simulink model "optotrak_double_pendulum_and_VR_v2"  (R2019b)
settings: Solver=ode3  StartTime=0.0  StopTime=inf  FixedStep=0.01  RelTol=1e-3  EnableMultiTasking=on
libraries: mblibv1 x4, xpcrtudplib x2, xpcutilitieslib x2, vrlib x2, slrtlib x1
(part 2 of 2)

== matlab function optotrak_double_pendulum_and_VR_v2/Embedded MATLAB Function1 ==
  data: R output; T1 input; T2 input
function R=R_iz_markerjev(T1,T2)
% Roman Kamnik, avgust 2010


%  Orientacijaska matrika segmenta iz markerjev.
%



%  H matrika pripeta na segment - lokalni ks
% osi koordinatenga sistema



tmp =  [0;0;1];
yos = unit(T1-T2);
xos = unit(cross(yos,tmp));
zos = unit(cross(xos, yos));

RR = [xos yos zos];

 
R = [RR(1,1); RR(2,1); RR(3,1); RR(1,2); RR(2,2); RR(3,2); RR(1,3); RR(2,3); RR(3,3)]; 
 
return;



%%%%%%%%%%%%%%%%%%%%%%%%%%%%%%%%%%%%%%%%%%%%%%%%%%%%%%%%%%%%%%%%%%%%%%%%

function u = unit(v)
	%u = v / norm(v,'fro');
    u = v / norm(v,2);
return    

% %%%%%%%%%%%%%%%%%%%%%%%%%%%%%%%%%%%%%%%%%%%%%%%%%%%%%%%%%%%%%%%%%%%%%%%%%

== matlab function optotrak_double_pendulum_and_VR_v2/Embedded MATLAB Function8 ==
  data: M1 input; COM output; M2 input
function COM= COM(M1, M2) 
% This block supports the Embedded MATLAB subset.
% See the help menu for details. 


d = 0.045;


C1 = M1;
C2 = M2;

COM = C1;



  
return;


%%%%%%%%%%%%%%%%%%%%%%%%%%%%%%%%%%%%%%%%%%%%%%%%%%%%%%%%%%%%%%%%%%%%%%%%

function u = unit(v)
	%u = v / norm(v,'fro');
    u = v / norm(v,2);
return    

% %%%%%%%%%%%%%%%%%%%%%%%%%%%%%%%%%%%%%%%%%%%%%%%%%%%%%%%%%%%%%%%%%%%%%%%%%

== matlab function optotrak_double_pendulum_and_VR_v2/Embedded MATLAB Function10 ==
  data: R1_in input size=[9 1]; X2 output; R2_in input size=[9 1]
function X2  = fcn1(R1_in,R2_in)
% This block supports the Embedded MATLAB subset.
% See the help menu for details. 


% Transformacija iz lokalnih ks segmentov v SimMech v lokalne ks segmentov v VR modelu
% columnwise as a 9-component row vector: (R11,  R21, R31,  R12, ... ).

% dolocitev orientacijske matrike med dvema segmentoma v vr, ce poznam R matriki v ks SimMech
% R1 je orientacija prvega segmenta, R2 drugega
% npr. R1 medenica, R2 thigh   ali pa R1 thigh in R2 shank
% X je orientacija glede na predhodni ks (VR)
% zasuk med ks segmenti in ks SimMech je roty(pi/2), zato je orientacija medenice kar roty(pi/2)
% X = inv(R1) * R2 * roty(pi/2)


%R_in = [ 1; 0; 0;  0; 1; 0;  0; 0; 1 ];   
%R_in = [ 1; 0; 0;  0; 0; -1;  0; 1; 0 ];   
%R1_in = [ 1; 0; 0;  0; 1; 0;  0; 0; 1 ];



R1_inn =[R1_in(1) R1_in(4) R1_in(7); ...
        R1_in(2) R1_in(5) R1_in(8); ...
        R1_in(3) R1_in(6) R1_in(9)] ;

%R1_inn = R1_inn * rotz(pi/2)    

%R2_in = [ 1; 0; 0;  0; 1; 0;  0; 0; 1 ];

R2_inn =[R2_in(1) R2_in(4) R2_in(7); ...
        R2_in(2) R2_in(5) R2_in(8); ...
        R2_in(3) R2_in(6) R2_in(9)] ;

%R2_inn = R2_inn * rotz(pi/3)    
    
    
   % X1 = inv(roty(pi/2))* R1_inn *roty(pi/2);  % orientacija 1. segmenta glede na ks medenice
   % X2 = inv(roty(pi/2))* R2_inn *roty(pi/2);  % orientacija 2. segmenta glede na ks medenice
   % RR = inv(X1)* X2;
   
   RR = inv(R1_inn)*R2_inn;
   
   
%RR = [unit(N(:)) unit(O(:)) unit(A(:))];  % dolocitev orientacijske R matrike segmenta

%R = [RR(1,1); RR(1,2); RR(1,3); RR(2,1); RR(2,2); RR(2,3); RR(3,1); RR(3,2); RR(3,3)];


X2 = [RR(1,1); RR(2,1); RR(3,1); RR(1,2); RR(2,2); RR(3,2); RR(1,3); RR(2,3); RR(3,3)];

%R =R_in;
%R = [RR(1); RR(2); RR(3); RR(4); RR(5); RR(6); RR(7); RR(8); RR(9)];


function u = unit(v)
	u = v / norm(v,'fro');
return    


function r = rotz(t)
	ct = cos(t);
	st = sin(t);
	r =    [ct	-st	0	
		st	ct	0	
		0	0	1	];
return

function r = rotx(t)
	ct = cos(t);
	st = sin(t);
	r =[1	0	0;...	
		0	ct	-st;...	
		0	st	ct	];
return    
    
function r = roty(t)
	ct = cos(t);
	st = sin(t);
	r =    [ct	0	st	
            0	1	0	
            -st	0	ct	];
return

== matlab function optotrak_double_pendulum_and_VR_v2/Embedded MATLAB Function7 ==
  data: R output; T1 input; T2 input
function R=R_iz_markerjev(T1,T2)
% Roman Kamnik, avgust 2010


%  Orientacijaska matrika segmenta iz markerjev.
%



%  H matrika pripeta na segment - lokalni ks
% osi koordinatenga sistema



tmp =  [0;0;1];
yos = unit(T1-T2);
xos = unit(cross(yos,tmp));
zos = unit(cross(xos, yos));

RR = [xos yos zos];

 
R = [RR(1,1); RR(2,1); RR(3,1); RR(1,2); RR(2,2); RR(3,2); RR(1,3); RR(2,3); RR(3,3)]; 
 
return;



%%%%%%%%%%%%%%%%%%%%%%%%%%%%%%%%%%%%%%%%%%%%%%%%%%%%%%%%%%%%%%%%%%%%%%%%

function u = unit(v)
	%u = v / norm(v,'fro');
    u = v / norm(v,2);
return    

% %%%%%%%%%%%%%%%%%%%%%%%%%%%%%%%%%%%%%%%%%%%%%%%%%%%%%%%%%%%%%%%%%%%%%%%%%

== matlab function optotrak_double_pendulum_and_VR_v2/Embedded MATLAB Function3 ==
  data: COM1 input; COM2 input; COM output
function COM= COM(COM1, COM2) 
% This block supports the Embedded MATLAB subset.
% See the help menu for details. 

m1 = 0.5;
m2 = 1.3;

;
COM = [0;0;0];


  
return;


%%%%%%%%%%%%%%%%%%%%%%%%%%%%%%%%%%%%%%%%%%%%%%%%%%%%%%%%%%%%%%%%%%%%%%%%

function u = unit(v)
	%u = v / norm(v,'fro');
    u = v / norm(v,2);
return    

% %%%%%%%%%%%%%%%%%%%%%%%%%%%%%%%%%%%%%%%%%%%%%%%%%%%%%%%%%%%%%%%%%%%%%%%%%

== matlab function optotrak_double_pendulum_and_VR_v2/Embedded MATLAB Function2 ==
  data: M1 input; COM output; M2 input
function COM= COM(M1, M2) 
% This block supports the Embedded MATLAB subset.
% See the help menu for details. 


d = 0.045;


C1 = M1;
C2 = M2;

COM = C1;



  
return;


%%%%%%%%%%%%%%%%%%%%%%%%%%%%%%%%%%%%%%%%%%%%%%%%%%%%%%%%%%%%%%%%%%%%%%%%

function u = unit(v)
	%u = v / norm(v,'fro');
    u = v / norm(v,2);
return    

% %%%%%%%%%%%%%%%%%%%%%%%%%%%%%%%%%%%%%%%%%%%%%%%%%%%%%%%%%%%%%%%%%%%%%%%%%

== matlab function optotrak_double_pendulum_and_VR_v2/OPTOTRAK Certus/Embedded MATLAB Function19 ==
  data: M_rot output; M input
function M_rot=rot_v_gl(M)
% Roman Kamnik, avgust 2010


%  ORotacija markerjev v globalni ks
% kot je pri veslanju



%  H matrika pripeta na segment - lokalni ks
% osi koordinatenga sistema

R = roty(pi/2)*rotx(pi/2);

 
M_rot = R * M(:) + [0.010125 ; 0.11977 ; 0.0];
 

%M_rot = M(:);
 
return;



%%%%%%%%%%%%%%%%%%%%%%%%%%%%%%%%%%%%%%%%%%%%%%%%%%%%%%%%%%%%%%%%%%%%%%%%

function u = unit(v)
	%u = v / norm(v,'fro');
    u = v / norm(v,2);
return    

% %%%%%%%%%%%%%%%%%%%%%%%%%%%%%%%%%%%%%%%%%%%%%%%%%%%%%%%%%%%%%%%%%%%%%%%%%
function r = rotz(t)
	ct = cos(t);
	st = sin(t);
	r =    [ct	-st	0	
		st	ct	0	
		0	0	1	];
return
% %%%%%%%%%%%%%%%%%%%%%%%%%%%%%%%%%%%%%%%%%%%%%%%%%%%%%%%%%%%%%%%%%%%%%%%%%

function r = rotx(t)
	ct = cos(t);
	st = sin(t);
	r =[1	0	0;...	
		0	ct	-st;...	
		0	st	ct	];
return    
  % %%%%%%%%%%%%%%%%%%%%%%%%%%%%%%%%%%%%%%%%%%%%%%%%%%%%%%%%%%%%%%%%%%%%%%%%%
  
function r = roty(t)
	ct = cos(t);
	st = sin(t);
	r =    [ct	0	st	
            0	1	0	
            -st	0	ct	];
return
% %%%%%%%%%%%%%%%%%%%%%%%%%%%%%%%%%%%%%%%%%%%%%%%%%%%%%%%%%%%%%%%%%%%%%%%%%
